simulink model "Electrical_Model"  (R2019a)
settings: Solver=VariableStepAuto  StartTime=0.0  StopTime=tFinal  RelTol=1e-3
libraries: powerlib x7, powerlib_meascontrol x3
settings Model: Creator=GKAR01  LastModifiedBy=GKAR01
settings SolverCC: ZeroCrossAlgorithm=Adaptive
settings DataIOCC: ReturnWorkspaceOutputs=off
settings DebuggingCC: IgnoredZcDiagnostic=none  UnconnectedInputMsg=none  UnconnectedOutputMsg=none  UnconnectedLineMsg=none  ArithmeticOperatorsInVariantConditions=warning
settings SFSimCC: SimUseLocalCustomCode=off
settings RTWCC: RTWUseLocalCustomCode=off
settings CodeAppCC: StateflowObjectComments=on
settings SimscapeCC: SimscapeNormalizeSystem=off

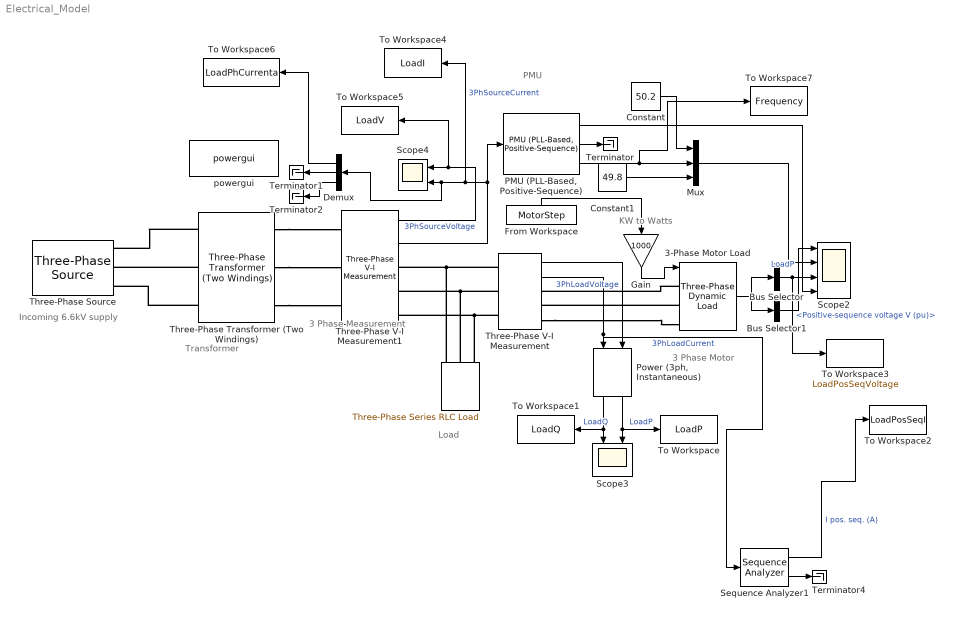
== system Electrical_Model ==
  note: PMU
  note: 3 Phase
      | Motor
  note: 3 Phase
      | Measurement
  note: Load
  note: Transformer
  note: KW to Watts
  note: Incoming
      | 6.6kV supply
  " " : powerlib/Elements/Three-Phase Series RLC Load  LConnTagsString=A|B|C  Configuration=Y (grounded)  NominalVoltage=400  Vabc=[1e3 1e3 1e3]  Vabcp=[1e3 1e3 1e3]  NominalFrequency=50  UnbalancedPower=off  ActivePower=5e3  InductivePower=0  CapacitivePower=0  Pabc=[10e3 9e3 11e3]  QLabc=[100 90 110]  QCabc=[100 90 110]  Pabcp=[10e3 9e3 11e3]  QLabcp=[100 90 110]  QCabcp=[100 90 110]  Measurements=None  LoadType=constant Z
      settings: SourceProductName=Simscape Electrical
  3-Phase Motor Load : powerlib/Elements/Three-Phase Dynamic Load  NominalVoltage=[ 400 50 ]  ActiveReactivePowers=[126843 63421.3]  PositiveSequence=[0.971714 -2.98544]  ExternalControl=on  NpNq="[1  1]"  TimeConstants="[0  0  0  0]"  MinimumVoltage=0.7  Tfilter=1e-4  LoadFlowParameters=[4 126842.66 0 0 63421.33]
      settings: SourceProductName=Simscape Electrical  SourceProductBaseCode=PS
  Bus Selector : BusSelector  OutputSignals=Positive-sequence voltage V (pu)
  Bus Selector1 : BusSelector  OutputSignals=Active power P (W)  OutputAsBus=on
  Constant : Constant  Value=50.2
  Constant1 : Constant  Value=49.8
  Demux : Demux  Outputs=3
  From Workspace : FromWorkspace  VariableName=MotorStep  SampleTime=0
  Gain : Gain  Gain=1000
  Mux : Mux  Inputs=3
  "PMU (PLL-Based, Positive-Sequence)" : powerlib_meascontrol/Measurements/PMU (PLL-Based, Positive-Sequence)  nominalFrequency=50  samplingRate=64  reportingFactor=1
      settings: SourceProductName=Simscape Electrical  SourceProductBaseCode=PS
  "Power (3ph, Instantaneous)" : powerlib_meascontrol/Measurements/Power (3ph, Instantaneous)
      settings: SourceProductName=Simscape Electrical
  Scope2 : Scope  NumInputPorts=4
  Scope3 : Scope  NumInputPorts=2
  Scope4 : Scope  NumInputPorts=2
  Sequence Analyzer1 : powerlib_meascontrol/Measurements/Sequence Analyzer  Freq=60  n=1  seq=Positive  InInit=[1, 0]  Ts=0
      settings: SourceProductName=Simscape Electrical  SourceProductBaseCode=PS
  Terminator{,1..2,4} (4 alike) : Terminator
  Three-Phase Transformer (Two Windings) : powerlib/Elements/Three-Phase Transformer (Two Windings)  Winding1Connection=Yg  Winding2Connection=Yg  CoreType=Three-limb core (core-type)  SetSaturation=off  Hysteresis=off  DataFile='hysteresis'  SetInitialFlux=off  Measurements=None  UNITS=pu  NominalPower=[ 400e3 , 50 ]  Winding1=[6600 0.002 0.066667]  Winding2=[400 0.0022222 0.088887]  Rm=555.56  Lm=555.55  L0=0.5  Saturation=[0 0;0.00216 1.2;0.9 1.52]  InitialFluxes=[ 0.8 , -0.8 , 0.7 ]  BreakLoop=off  DiscreteSolver=Trapezoidal iterative  DataType=off  TransfoNumber=1
      settings: SourceProductName=Simscape Electrical
  Three-Phase V-I Measurement : powerlib/Measurements/Three-Phase V-I Measurement  VoltageMeasurement=phase-to-ground  SetLabelV=off  LabelV=V1  Vpu=off  VpuLL=off  CurrentMeasurement=yes  SetLabelI=off  LabelI=I1  Ipu=off  Pbase=100e6  Vbase=500e3  OutputType=Magnitude  PhasorSimulation=off  PSBequivalent=0
      settings: SourceProductName=Simscape Electrical
  Three-Phase V-I Measurement1 : powerlib/Measurements/Three-Phase V-I Measurement  VoltageMeasurement=phase-to-ground  SetLabelV=off  LabelV=V1  Vpu=off  VpuLL=off  CurrentMeasurement=yes  SetLabelI=off  LabelI=I1  Ipu=off  Pbase=100e6  Vbase=500e3  OutputType=Magnitude  PhasorSimulation=off  PSBequivalent=0
      settings: SourceProductName=Simscape Electrical
  Three-Phase Source : powerlib/Electrical Sources/Three-Phase Source  InternalConnection=Yg  VoltagePhases=off  Voltage=(6600)*1  PhaseAngle=0  Voltage_phases=[25e3 25e3 25e3]/sqrt(3)  PhaseAngles_phases=[0 -120 +120]  Frequency=50  NonIdealSource=off  SpecifyImpedance=off  Resistance=0.8929  Inductance=16.58e-3  ShortCircuitLevel=100e6  BaseVoltage=6.6e3  XRratio=7  BusType=swing  Pref=20e6  Qref=0  Prefabc=[10e3, 10e3, 10e3]  Qrefabc=[0, 0, 0]  Qmin=-inf  Qmax=inf
      settings: SourceProductName=Simscape Electrical
  To Workspace : ToWorkspace  VariableName=LoadP  SaveFormat=Structure With Time  SampleTime=-1
  To Workspace1 : ToWorkspace  VariableName=LoadQ  SaveFormat=Structure With Time  SampleTime=-1
  To Workspace2 : ToWorkspace  VariableName=LoadPosSeqI  SaveFormat=Structure With Time  SampleTime=-1
  To Workspace3 : ToWorkspace  VariableName=LoadPosSeqVoltage  SaveFormat=Structure With Time  SampleTime=-1
  To Workspace4 : ToWorkspace  VariableName=LoadI  SaveFormat=Structure With Time  SampleTime=-1
  To Workspace5 : ToWorkspace  VariableName=LoadV  SaveFormat=Structure With Time  SampleTime=-1
  To Workspace6 : ToWorkspace  VariableName=LoadPhCurrenta  SaveFormat=Structure With Time  SampleTime=-1
  To Workspace7 : ToWorkspace  VariableName=Frequency  SaveFormat=Structure With Time  SampleTime=-1
  powergui : powerlib/powergui  Priority=2  SimulationMode=Continuous  SampleTime=1  frequency=60  Iterations=50  frequencyindice=50  Pbase=100e6  ErrMax=0.0001  UnitsV=kV  UnitsW=MW  buscounter=0  FunctionMessages=off  echomessages=off  EnableUseOfTLC=off  CurrentSourceSwitches=on  DisableSnubberDevices=off  DisableRonSwitches=off  DisableVfSwitches=off  DisplayEquations=off  AutomaticDiscreteSolvers=off  SolverType=Tustin  Interpol=off  ExternalGateDelay=off  methode=off  Ts=0  x0status=blocks  SPID=off  SwTol=0  HookPort=off  NonlinearTolerance=0  nMaxIteration=15  ContinueOnMaxIteration=off  RestoreLinks=warning  ResistiveCurrentMeasurement=off  Frange=[0:2:500]  Ylog=off  Xlog=off  ShowGrid=off  save=off  variable=ZData  structure=0  ZoomFFT=on  StartTime=0.0  cycles=1  DisplayStyle=off  fundamental=60  FreqAxis=off  MaxFrequency=1000  frequencyindicesteady=1  RmsSteady=2  display=off
      settings: SourceProductName=Simscape Electrical
  wires:
  Gain/1 -> 3-Phase Motor Load/1
  Three-Phase V-I Measurement1/1 -> To Workspace5/1, Scope4/1  "3PhSourceVoltage"
  "PMU (PLL-Based, Positive-Sequence)"/1 -> Scope2/4
  "PMU (PLL-Based, Positive-Sequence)"/2 -> Terminator/1
  Three-Phase V-I Measurement1/2 -> "PMU (PLL-Based, Positive-Sequence)"/1, To Workspace4/1, Demux/1, Scope4/2  "3PhSourceCurrent"
  3-Phase Motor Load/1 -> Bus Selector/1, Bus Selector1/1
  Three-Phase V-I Measurement/2 -> Sequence Analyzer1/1, "Power (3ph, Instantaneous)"/2  "3PhLoadCurrent"
  Three-Phase V-I Measurement/1 -> "Power (3ph, Instantaneous)"/1  "3PhLoadVoltage"
  Bus Selector/1 -> To Workspace3/1, Scope2/3  "<Positive-sequence voltage V (pu)>"
  Bus Selector1/1 -> Scope2/1  "LoadP"
  From Workspace/1 -> Gain/1
  "Power (3ph, Instantaneous)"/2 -> To Workspace1/1, Scope3/1  "LoadQ"
  "Power (3ph, Instantaneous)"/1 -> To Workspace/1, Scope3/2  "LoadP"
  "PMU (PLL-Based, Positive-Sequence)"/3 -> To Workspace7/1, Mux/2
  Mux/1 -> Scope2/2
  Constant1/1 -> Mux/3
  Constant/1 -> Mux/1
  Demux/1 -> To Workspace6/1
  Demux/2 -> Terminator1/1
  Demux/3 -> Terminator2/1
  Sequence Analyzer1/1 -> To Workspace2/1  "I pos. seq. (A)"
  Sequence Analyzer1/2 -> Terminator4/1
  connections:
  Three-Phase Transformer (Two Windings)/LConn1 -- Three-Phase Source/RConn1
  Three-Phase Transformer (Two Windings)/LConn2 -- Three-Phase Source/RConn2
  Three-Phase Transformer (Two Windings)/RConn1 -- Three-Phase V-I Measurement1/LConn1
  Three-Phase Transformer (Two Windings)/RConn2 -- Three-Phase V-I Measurement1/LConn2
  Three-Phase Transformer (Two Windings)/RConn3 -- Three-Phase V-I Measurement1/LConn3
  Three-Phase Transformer (Two Windings)/LConn3 -- Three-Phase Source/RConn3
  Three-Phase V-I Measurement/LConn1 -- " "/LConn1 -- Three-Phase V-I Measurement1/RConn1
  Three-Phase V-I Measurement/LConn2 -- " "/LConn2 -- Three-Phase V-I Measurement1/RConn2
  Three-Phase V-I Measurement/LConn3 -- " "/LConn3 -- Three-Phase V-I Measurement1/RConn3
  3-Phase Motor Load/LConn2 -- Three-Phase V-I Measurement/RConn2
  3-Phase Motor Load/LConn1 -- Three-Phase V-I Measurement/RConn1
  Three-Phase V-I Measurement/RConn3 -- 3-Phase Motor Load/LConn3
